simulink model "ex3S"  (R2022a)
settings: Solver=VariableStepAuto  StartTime=0.0  StopTime=10.0  RelTol=1e-3
settings Model: Creator=Guilherme  LastModifiedBy=Guilherme

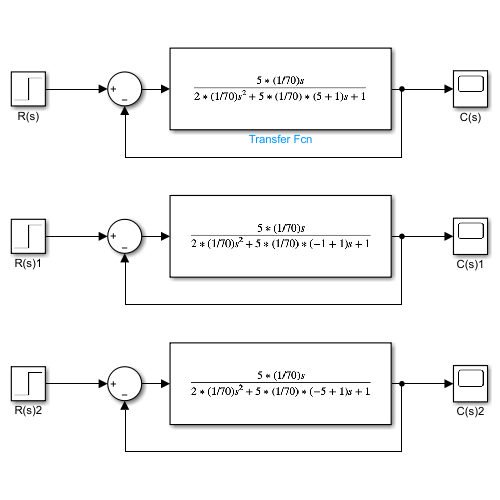
[thumbnail: Simulink's stored preview of the top-level diagram]
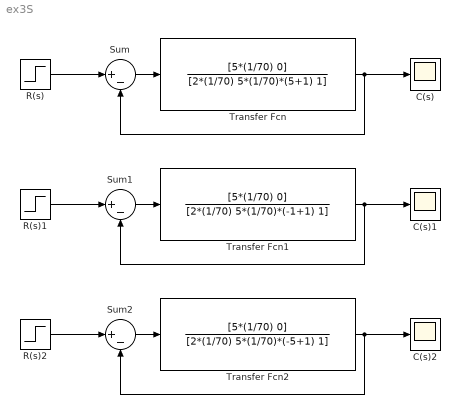
== system ex3S ==
  C(s) : Scope
  C(s)1 : Scope
  C(s)2 : Scope
  R(s) : Step  Time=0  SampleTime=0
  R(s)1 : Step  Time=0  SampleTime=0
  R(s)2 : Step  Time=0  SampleTime=0
  Sum : Sum  Inputs=|+-
  Sum1 : Sum  Inputs=|+-
  Sum2 : Sum  Inputs=|+-
  Transfer Fcn : TransferFcn  Numerator=[5*(1/70) 0]  Denominator=[2*(1/70) 5*(1/70)*(5+1) 1]
  Transfer Fcn1 : TransferFcn  Numerator=[5*(1/70) 0]  Denominator=[2*(1/70) 5*(1/70)*(-1+1) 1]
  Transfer Fcn2 : TransferFcn  Numerator=[5*(1/70) 0]  Denominator=[2*(1/70) 5*(1/70)*(-5+1) 1]
  wires:
  Transfer Fcn/1 -> C(s)/1, Sum/2
  R(s)/1 -> Sum/1
  Sum/1 -> Transfer Fcn/1
  Transfer Fcn1/1 -> C(s)1/1, Sum1/2
  R(s)1/1 -> Sum1/1
  Sum1/1 -> Transfer Fcn1/1
  Transfer Fcn2/1 -> C(s)2/1, Sum2/2
  R(s)2/1 -> Sum2/1
  Sum2/1 -> Transfer Fcn2/1
